simulink model "ims_Build5pt1g_tj"  (R2020b)
settings: Solver=FixedStepDiscrete  StartTime=0.0  StopTime=180  FixedStep=fem.Ts  RelTol=1e-4
InitFcn:
  | %
  | % Initialization callback function
  | %
  | 
  | try
  |    fprintf('\n New GMT IMS version!\n');
  | 
  |    % Get Simulink model directory
  |    [filepath,name,ext] = fileparts(which(bdroot));
  | 
  |    if ~strcmp(filepath,pwd)
  |       fprintf('\n Changing current directory to \n %s \n',filepath);
  |       cd(filepath);
  |    end
  | 
  |    %
  |    if(~exist('IMLoads','var'))
  |        warning('Simulation model assumes wind load is loaded...');
  |    end
  | catch
  |    warning('Running the InitFcn from puSimulate script');
  | end
values from neighbouring files (symbols this model uses):
  az = zeros(N,1)    [eval_trajectories.m]
  az_ff_en = 1    [load_IMS_5pt1g_tj.m]    (also in load_IMS_5pt1h_tj.m = 0)
  el = az    [eval_trajectories.m]
  el_ff_en = 1    [load_IMS_5pt1g_tj.m]    (also in load_IMS_5pt1h_tj.m = 0)
  fem =     [controls_5pt1g1K_z00_llTT_oad.mat]    (also in controls_5pt1g1K_z30_llTT_oad.mat)
  FEM_Ts = 1/1e3    (= 0.001)    [load_IMS_5pt1g_tj.m]    (also in load_IMS_5pt1h_tj.m)
  gir = az    [eval_trajectories.m]
  gir_ff_en = 1    [load_IMS_5pt1g_tj.m]    (also in load_IMS_5pt1h_tj.m = 0)
  H_tj = tf(1,[2*pi*0.1, 1])    [eval_trajectories.m]    (also in load_IMS_5pt1g_tj.m = c2d(Htjf,FEM_Ts, 'foh'); load_IMS_5pt1h_tj.m = c2d(Htjf,FEM_Ts, 'foh'))
  Hkin_fsm = Phi(fsm_out,1:3) * Phi_mnt_pinv    [compute_Hkin.m]
  Hkin_hp = Phi(hp_out,1:3) * Phi_mnt_pinv    [compute_Hkin.m]
  Hkin_m12 = [Phi(m1_out,1:3); Phi(m2_out,1:3)] * Phi_mnt_pinv    [compute_Hkin.m]    (also in eval_tjs.m = [Phi(m1_out,1:3); Phi(m2_out,1:3)] * pinv(Phi_mnt_enc))
  Hkin_m2p = Phi(m2p_out,1:3) * Phi_mnt_pinv    [compute_Hkin.m]
  Hkin_pmtnodes = Phi(pmt_out,1:3) * Phi_mnt_pinv    [compute_Hkin.m]    (also in eval_tjs.m = Phi(pmt_out,1:3) * pinv(Phi_mnt_enc))
  m1olf_en = 0    [load_IMS_5pt1g_tj.m]    (also in load_IMS_5pt1h_tj.m)
  m1sys =     [controls_5pt1g1K_z00_llTT_oad.mat]    (also in controls_5pt1g1K_z30_llTT_oad.mat)
  m2_pos_en = 0    [load_IMS_5pt1g_tj.m]    (also in load_IMS_5pt1h_tj.m)
  m2pos =     [controls_5pt1g1K_z00_llTT_oad.mat]    (also in controls_5pt1g1K_z30_llTT_oad.mat)
  m2pzt =     [controls_5pt1g1K_z00_llTT_oad.mat]    (also in controls_5pt1g1K_z30_llTT_oad.mat)
  m2PZT_en = 0    [load_IMS_5pt1g_tj.m]    (also in load_IMS_5pt1h_tj.m)
  mntFBc_en = 1    [load_IMS_5pt1g_tj.m]    (also in load_IMS_5pt1h_tj.m)
  mount =     [controls_5pt1g1K_z00_llTT_oad.mat]    (also in controls_5pt1g1K_z30_llTT_oad.mat; eval_tjs.m = mountY)
  om2 = (2*pi*eigenfrequencies).^2    [load_IMS_5pt1g_tj.m]    (also in load_IMS_5pt1h_tj.m)
  PG = zeros(length(om2),6)    [load_IMS_5pt1g_tj.m]    (also in load_IMS_5pt1h_tj.m)
  phiB = Phim(indDesInputs,:)'    [load_IMS_5pt1g_tj.m]    (also in load_IMS_5pt1h_tj.m)
  phiC = Phi(indDesOutputs,:)    [load_IMS_5pt1g_tj.m]    (also in load_IMS_5pt1h_tj.m)
  pmt1 = dlmread(pmt1_fname,',',[14,3,27,302])    [eval_tjs.m]    (also in eval_tjs_rtf_variants.m; load_IMS_5pt1g_tj.m; load_IMS_5pt1h_tj.m)
  pmt2 = dlmread(pmt2_fname,',',[14,3,10,302])    [eval_tjs.m]    (also in eval_tjs_rtf_variants.m; load_IMS_5pt1g_tj.m; load_IMS_5pt1h_tj.m)
  Psi_ss = gainMatrix(indDesOutputs,indDesInputs) - K_ss    [load_IMS_5pt1g_tj.m]    (also in load_IMS_5pt1h_tj.m)
  Psi_ssTs = 1/1000    (= 0.001)    [load_IMS_5pt1g_tj.m]    (also in load_IMS_5pt1h_tj.m)
  twice_zom = adjDamp*twice_zom    [load_IMS_5pt1g_tj.m]    (also in load_IMS_5pt1h_tj.m)
undefined symbols (not defined in the file or in its folder): DiscIntNeverNeededParam, magnitude
libraries: ims_block_library x20, simulink x1
(part 2 of 2)

== system ims_Build5pt1g_tj/M2_PZT_Control/PZT_Control_FSM3 ==
  PZT_cmd : Inport
  PZT_FB : Inport  Port=2
  Sum : Sum  Inputs=|+-
  multi-rate SS : ims_block_library/multi-rate SS  ss_model=m2pzt{3}.SSdtHfb
  rel_PZT_D : Gain  Gain=kron(eye(3),[-1,1])  Multiplication=Matrix(K*u)
  spliF_matrix : Gain  Gain=kron(eye(3),[-1;1])  Multiplication=Matrix(K*u)
  m2PZT_u : Outport  VectorParamsAs1DForOutWhenUnconnected=off
  wires:
  Sum/1 -> multi-rate SS/1
  spliF_matrix/1 -> m2PZT_u/1
  PZT_FB/1 -> rel_PZT_D/1
  rel_PZT_D/1 -> Sum/2
  PZT_cmd/1 -> Sum/1
  multi-rate SS/1 -> spliF_matrix/1

== system ims_Build5pt1g_tj/M2_PZT_Control/PZT_Control_FSM4 ==
  PZT_cmd : Inport
  PZT_FB : Inport  Port=2
  Sum : Sum  Inputs=|+-
  multi-rate SS : ims_block_library/multi-rate SS  ss_model=m2pzt{4}.SSdtHfb
  rel_PZT_D : Gain  Gain=kron(eye(3),[-1,1])  Multiplication=Matrix(K*u)
  spliF_matrix : Gain  Gain=kron(eye(3),[-1;1])  Multiplication=Matrix(K*u)
  m2PZT_u : Outport  VectorParamsAs1DForOutWhenUnconnected=off
  wires:
  Sum/1 -> multi-rate SS/1
  spliF_matrix/1 -> m2PZT_u/1
  PZT_FB/1 -> rel_PZT_D/1
  rel_PZT_D/1 -> Sum/2
  PZT_cmd/1 -> Sum/1
  multi-rate SS/1 -> spliF_matrix/1

== system ims_Build5pt1g_tj/M2_PZT_Control/PZT_Control_FSM5 ==
  PZT_cmd : Inport
  PZT_FB : Inport  Port=2
  Sum : Sum  Inputs=|+-
  multi-rate SS : ims_block_library/multi-rate SS  ss_model=m2pzt{5}.SSdtHfb
  rPZT : Scope
  rel_PZT_D : Gain  Gain=kron(eye(3),[-1,1])  Multiplication=Matrix(K*u)
  spliF_matrix : Gain  Gain=kron(eye(3),[-1;1])  Multiplication=Matrix(K*u)
  m2PZT_u : Outport  VectorParamsAs1DForOutWhenUnconnected=off
  wires:
  Sum/1 -> rPZT/1, multi-rate SS/1
  spliF_matrix/1 -> m2PZT_u/1
  PZT_FB/1 -> rel_PZT_D/1
  rel_PZT_D/1 -> Sum/2
  PZT_cmd/1 -> Sum/1
  multi-rate SS/1 -> spliF_matrix/1

== system ims_Build5pt1g_tj/M2_PZT_Control/PZT_Control_FSM6 ==
  PZT_cmd : Inport
  PZT_FB : Inport  Port=2
  Sum : Sum  Inputs=|+-
  multi-rate SS : ims_block_library/multi-rate SS  ss_model=m2pzt{6}.SSdtHfb
  rel_PZT_D : Gain  Gain=kron(eye(3),[-1,1])  Multiplication=Matrix(K*u)
  spliF_matrix : Gain  Gain=kron(eye(3),[-1;1])  Multiplication=Matrix(K*u)
  m2PZT_u : Outport  VectorParamsAs1DForOutWhenUnconnected=off
  wires:
  Sum/1 -> multi-rate SS/1
  spliF_matrix/1 -> m2PZT_u/1
  PZT_FB/1 -> rel_PZT_D/1
  rel_PZT_D/1 -> Sum/2
  PZT_cmd/1 -> Sum/1
  multi-rate SS/1 -> spliF_matrix/1

== system ims_Build5pt1g_tj/M2_PZT_Control/PZT_Control_FSM7 ==
  PZT_cmd : Inport
  PZT_FB : Inport  Port=2
  Sum : Sum  Inputs=|+-
  multi-rate SS : ims_block_library/multi-rate SS  ss_model=m2pzt{7}.SSdtHfb
  rel_PZT_D : Gain  Gain=kron(eye(3),[-1,1])  Multiplication=Matrix(K*u)
  spliF_matrix : Gain  Gain=kron(eye(3),[-1;1])  Multiplication=Matrix(K*u)
  m2PZT_u : Outport  VectorParamsAs1DForOutWhenUnconnected=off
  wires:
  Sum/1 -> multi-rate SS/1
  spliF_matrix/1 -> m2PZT_u/1
  PZT_FB/1 -> rel_PZT_D/1
  rel_PZT_D/1 -> Sum/2
  PZT_cmd/1 -> Sum/1
  multi-rate SS/1 -> spliF_matrix/1

== system ims_Build5pt1g_tj/Mount_Drv_PDR2021/AZ DT Lugre Fr model ==
  vel : Inport
  Enable : EnablePort
  Constant : Constant  Value=frParStruct.iIsSig01Active
  Discrete-Time Integrator : DiscreteIntegrator  SampleTime=-1  ICPrevOutput=DiscIntNeverNeededParam  ICPrevScaledInput=DiscIntNeverNeededParam
  Sum : Sum  Inputs=+++
  g(v) : Subsystem
  sigma_0 : Gain  Gain=frParStruct.sigm0
  sigma_1 : Gain  Gain=frParStruct.sigm1
  sigma_v : Gain  Gain=frParStruct.sigmv
  v2z : Subsystem
  FrTorque : Outport  VectorParamsAs1DForOutWhenUnconnected=off
  wires:
  Discrete-Time Integrator/1 -> sigma_0/1, v2z/3(z)
  g(v)/1(g) -> v2z/2(g(v))
  sigma_v/1 -> Sum/3  "Viscose Friction"
  v2z/1(dz) -> Discrete-Time Integrator/1, sigma_1/1
  sigma_1/1 -> Sum/1
  sigma_0/1 -> Sum/2
  Sum/1 -> FrTorque/1
  vel/1 -> v2z/1(v), g(v)/1(v), sigma_v/1
  Constant/1 -> g(v)/Enable, v2z/Enable

== system ims_Build5pt1g_tj/Mount_Drv_PDR2021/EL DT Lugre Fr model ==
  vel : Inport
  Enable : EnablePort
  Constant : Constant  Value=frParStruct.iIsSig01Active
  Discrete-Time Integrator : DiscreteIntegrator  SampleTime=-1  ICPrevOutput=DiscIntNeverNeededParam  ICPrevScaledInput=DiscIntNeverNeededParam
  Sum : Sum  Inputs=+++
  To Workspace : ToWorkspace  VariableName=el_Ve  SampleTime=-1
  To Workspace1 : ToWorkspace  VariableName=el_To  SampleTime=-1
  g(v) : Subsystem
  sigma_0 : Gain  Gain=frParStruct.sigm0
  sigma_1 : Gain  Gain=frParStruct.sigm1
  sigma_v : Gain  Gain=frParStruct.sigmv
  v2z : Subsystem
  FrTorque : Outport  VectorParamsAs1DForOutWhenUnconnected=off
  wires:
  sigma_v/1 -> Sum/3  "Viscose Friction"
  vel/1 -> v2z/1(v), g(v)/1(v), To Workspace/1, sigma_v/1
  Constant/1 -> g(v)/Enable, v2z/Enable
  sigma_0/1 -> Sum/2
  g(v)/1(g) -> v2z/2(g(v))
  sigma_1/1 -> Sum/1
  Discrete-Time Integrator/1 -> sigma_0/1, v2z/3(z)
  v2z/1(dz) -> Discrete-Time Integrator/1, sigma_1/1
  Sum/1 -> To Workspace1/1, FrTorque/1

== system ims_Build5pt1g_tj/Mount_Drv_PDR2021/GIR DT Lugre Fr model ==
  vel : Inport
  Enable : EnablePort
  Discrete-Time Integrator : DiscreteIntegrator  SampleTime=-1  ICPrevOutput=DiscIntNeverNeededParam  ICPrevScaledInput=DiscIntNeverNeededParam
  Gain : Gain  Gain=frParStruct.iIsSig01Active
  Scope : Scope
  Sum : Sum  Inputs=+++
  To Workspace : ToWorkspace  VariableName=gir_Ve  SampleTime=-1
  To Workspace1 : ToWorkspace  VariableName=gir_To  SampleTime=-1
  g(v) : Subsystem
  sigma_0 : Gain  Gain=frParStruct.sigm0
  sigma_1 : Gain  Gain=frParStruct.sigm1
  sigma_v : Gain  Gain=frParStruct.sigmv
  v2z : Subsystem
  FrTorque : Outport  VectorParamsAs1DForOutWhenUnconnected=off
  wires:
  sigma_v/1 -> Sum/3  "Viscose Friction"
  vel/1 -> Gain/1, To Workspace/1, sigma_v/1
  sigma_0/1 -> Sum/2
  g(v)/1(g) -> v2z/2(g(v))
  Discrete-Time Integrator/1 -> sigma_0/1, v2z/3(z)
  v2z/1(dz) -> Discrete-Time Integrator/1, Scope/1, sigma_1/1
  Sum/1 -> To Workspace1/1, FrTorque/1
  sigma_1/1 -> Sum/1
  Gain/1 -> v2z/1(v), g(v)/1(v)

== system ims_Build5pt1g_tj/Mount_Drv_PDR2021/ODC CT LUGRE Fr model ==
  Az vel : Inport
  EL_vel : Inport  Port=2
  GIR vel : Inport  Port=3
  Constant2 : Constant
  Demux1 : Demux  Outputs=3
  Friction : Subsystem
  Mux7 : Mux  Inputs=3
  Az Fr To : Outport  VectorParamsAs1DForOutWhenUnconnected=off
  El Fr To : Outport  Port=2  VectorParamsAs1DForOutWhenUnconnected=off
  Gir Fr To : Outport  Port=3  VectorParamsAs1DForOutWhenUnconnected=off
  wires:
  Mux7/1 -> Friction/1(Vel)
  Demux1/2 -> El Fr To/1
  Demux1/1 -> Az Fr To/1
  Friction/1(FrictionTo) -> Demux1/1
  Constant2/1 -> Friction/Enable
  Demux1/3 -> Gir Fr To/1
  Az vel/1 -> Mux7/1
  EL_vel/1 -> Mux7/2
  GIR vel/1 -> Mux7/3

== system ims_Build5pt1g_tj/Mount_Drv_PDR2021/Parasitic torques model  ==
  Az_pos_drv : Inport
  El_pos_drv : Inport  Port=2
  Gir_pos_drv : Inport  Port=3
  Az_drv_to : Inport  Port=4
  El_drv_to : Inport  Port=5
  Gir_drv_to : Inport  Port=6
  AZ_Parasitic_Torque : Subsystem  mask{ParasiticModelStruc=mount.az.ParasiticTo}
      mask prompts: ParasiticModelStruc "Parasitic Torque Model Parameters Structure"
  EL_Parasitic_Torque : Subsystem  mask{ParasiticModelStruc=mount.el.ParasiticTo}
      mask prompts: ParasiticModelStruc "Parasitic Torque Model Parameters Structure"
  GIR_Parasitic_Torque : Subsystem  mask{ParasiticModelStruc=mount.gir.ParasiticTo, T_pretension=mount.gir.T_pretension}
      mask prompts: ParasiticModelStruc "Parasitic Torque Model Parameters Structure"; T_pretension "Pretension torque"
  Mux1 : Mux  Commented=on  Inputs=2
  Mux2 : Mux  Commented=on  Inputs=2
  Mux6 : Mux  Commented=on  Inputs=2
  ParTo_Scope : Scope  Commented=on  NumInputPorts=3
  Subsystem : Subsystem  Commented=on
  Az_Par_To : Outport  VectorParamsAs1DForOutWhenUnconnected=off
  El_Par_To : Outport  Port=2  VectorParamsAs1DForOutWhenUnconnected=off
  Gir_Par_To : Outport  Port=3  VectorParamsAs1DForOutWhenUnconnected=off
  wires:
  Az_drv_to/1 -> Subsystem/2(Az To), AZ_Parasitic_Torque/2(Drive_Torque)
  Gir_drv_to/1 -> Subsystem/6(Gir To), GIR_Parasitic_Torque/2(Drive_Torque)
  GIR_Parasitic_Torque/1(Parasitic_Torque) -> Gir_Par_To/1, Mux6/1
  Gir_pos_drv/1 -> Subsystem/5(Gir Pos), GIR_Parasitic_Torque/1(Drive_Pos)
  El_drv_to/1 -> Subsystem/4(El To), EL_Parasitic_Torque/2(Drive_Torque)
  Az_pos_drv/1 -> Subsystem/1(Az Pos), AZ_Parasitic_Torque/1(Drive_Pos)
  El_pos_drv/1 -> Subsystem/3(El Pos), EL_Parasitic_Torque/1(Drive_Pos)
  AZ_Parasitic_Torque/1(Parasitic_Torque) -> Mux2/1, Az_Par_To/1
  EL_Parasitic_Torque/1(Parasitic_Torque) -> El_Par_To/1, Mux1/1
  Mux2/1 -> ParTo_Scope/1
  Mux1/1 -> ParTo_Scope/2
  Mux6/1 -> ParTo_Scope/3
  Subsystem/1(Out1) -> Mux2/2
  Subsystem/2(Out2) -> Mux1/2
  Subsystem/3(Out3) -> Mux6/2

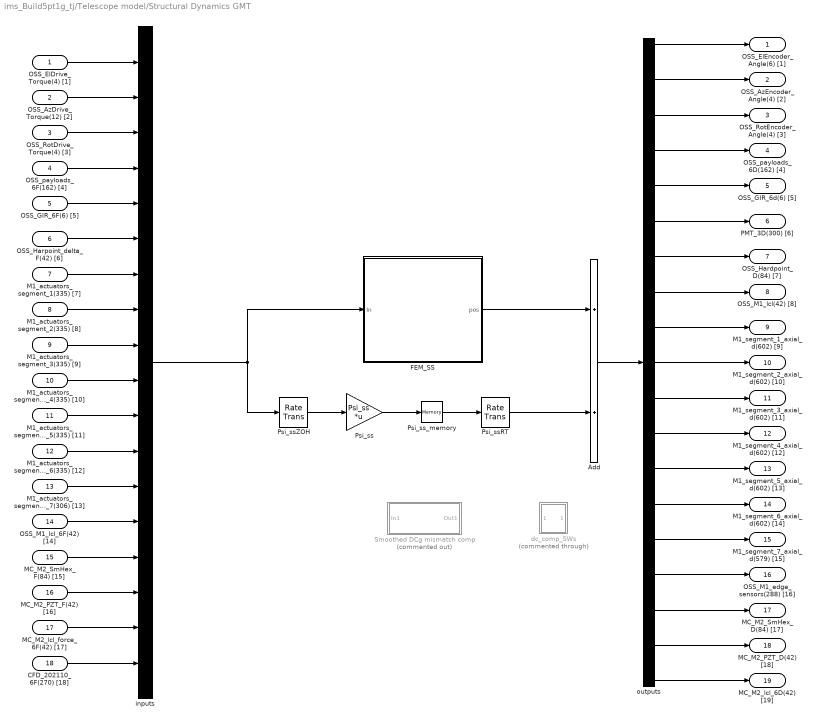
== system ims_Build5pt1g_tj/Telescope model/Structural Dynamics GMT ==
  OSS_ElDrive_Torque(4) [1] : Inport  PortDimensions=4
  OSS_AzDrive_Torque(12) [2] : Inport  Port=2  PortDimensions=12
  OSS_RotDrive_Torque(4) [3] : Inport  Port=3  PortDimensions=4
  OSS_payloads_6F(162) [4] : Inport  Port=4  PortDimensions=162
  OSS_GIR_6F(6) [5] : Inport  Port=5  PortDimensions=6
  OSS_Harpoint_delta_F(42) [6] : Inport  Port=6  PortDimensions=42
  M1_actuators_segment_1(335) [7] : Inport  Port=7  PortDimensions=335
  M1_actuators_segment_2(335) [8] : Inport  Port=8  PortDimensions=335
  M1_actuators_segment_3(335) [9] : Inport  Port=9  PortDimensions=335
  M1_actuators_segment_4(335) [10] : Inport  Port=10  PortDimensions=335
  M1_actuators_segment_5(335) [11] : Inport  Port=11  PortDimensions=335
  M1_actuators_segment_6(335) [12] : Inport  Port=12  PortDimensions=335
  M1_actuators_segment_7(306) [13] : Inport  Port=13  PortDimensions=306
  OSS_M1_lcl_6F(42) [14] : Inport  Port=14  PortDimensions=42
  MC_M2_SmHex_F(84) [15] : Inport  Port=15  PortDimensions=84
  MC_M2_PZT_F(42) [16] : Inport  Port=16  PortDimensions=42
  MC_M2_lcl_force_6F(42) [17] : Inport  Port=17  PortDimensions=42
  CFD_202110_6F(270) [18] : Inport  Port=18  PortDimensions=270
  Add : Sum
  FEM_SS : Subsystem
  Psi_ss : Gain  Gain=Psi_ss  Multiplication=Matrix(K*u) (u vector)
  Psi_ssRT : RateTransition  Deterministic=off  OutPortSampleTimeOpt=Inherit
  Psi_ssZOH : RateTransition  Deterministic=off  OutPortSampleTime=Psi_ssTs
  Psi_ss_memory : Memory  InitialCondition=zeros(size(phiC,1),1)  InheritSampleTime=on  LinearizeAsDelay=on
  Smoothed DCg mismatch comp : Subsystem  Commented=on
  dc_comp_SWs : Subsystem  Commented=through
  inputs : Mux  Inputs=modelMuxDims
  outputs : Demux  Outputs=modelDemuxDims
  OSS_ElEncoder_Angle(6) [1] : Outport  PortDimensions=6  VectorParamsAs1DForOutWhenUnconnected=off
  OSS_AzEncoder_Angle(4) [2] : Outport  Port=2  PortDimensions=4  VectorParamsAs1DForOutWhenUnconnected=off
  OSS_RotEncoder_Angle(4) [3] : Outport  Port=3  PortDimensions=4  VectorParamsAs1DForOutWhenUnconnected=off
  OSS_payloads_6D(162) [4] : Outport  Port=4  PortDimensions=162  VectorParamsAs1DForOutWhenUnconnected=off
  OSS_GIR_6d(6) [5] : Outport  Port=5  PortDimensions=6  VectorParamsAs1DForOutWhenUnconnected=off
  PMT_3D(300) [6] : Outport  Port=6  PortDimensions=300  VectorParamsAs1DForOutWhenUnconnected=off
  OSS_Hardpoint_D(84) [7] : Outport  Port=7  PortDimensions=84  VectorParamsAs1DForOutWhenUnconnected=off
  OSS_M1_lcl(42) [8] : Outport  Port=8  PortDimensions=42  VectorParamsAs1DForOutWhenUnconnected=off
  M1_segment_1_axial_d(602) [9] : Outport  Port=9  PortDimensions=602  VectorParamsAs1DForOutWhenUnconnected=off
  M1_segment_2_axial_d(602) [10] : Outport  Port=10  PortDimensions=602  VectorParamsAs1DForOutWhenUnconnected=off
  M1_segment_3_axial_d(602) [11] : Outport  Port=11  PortDimensions=602  VectorParamsAs1DForOutWhenUnconnected=off
  M1_segment_4_axial_d(602) [12] : Outport  Port=12  PortDimensions=602  VectorParamsAs1DForOutWhenUnconnected=off
  M1_segment_5_axial_d(602) [13] : Outport  Port=13  PortDimensions=602  VectorParamsAs1DForOutWhenUnconnected=off
  M1_segment_6_axial_d(602) [14] : Outport  Port=14  PortDimensions=602  VectorParamsAs1DForOutWhenUnconnected=off
  M1_segment_7_axial_d(579) [15] : Outport  Port=15  PortDimensions=579  VectorParamsAs1DForOutWhenUnconnected=off
  OSS_M1_edge_sensors(288) [16] : Outport  Port=16  PortDimensions=288  VectorParamsAs1DForOutWhenUnconnected=off
  MC_M2_SmHex_D(84) [17] : Outport  Port=17  PortDimensions=84  VectorParamsAs1DForOutWhenUnconnected=off
  MC_M2_PZT_D(42) [18] : Outport  Port=18  PortDimensions=42  VectorParamsAs1DForOutWhenUnconnected=off
  MC_M2_lcl_6D(42) [19] : Outport  Port=19  PortDimensions=42  VectorParamsAs1DForOutWhenUnconnected=off
  wires:
  outputs/19 -> MC_M2_lcl_6D(42) [19]/1
  outputs/18 -> MC_M2_PZT_D(42) [18]/1
  outputs/17 -> MC_M2_SmHex_D(84) [17]/1
  outputs/16 -> OSS_M1_edge_sensors(288) [16]/1
  outputs/15 -> M1_segment_7_axial_d(579) [15]/1
  outputs/14 -> M1_segment_6_axial_d(602) [14]/1
  outputs/13 -> M1_segment_5_axial_d(602) [13]/1
  outputs/12 -> M1_segment_4_axial_d(602) [12]/1
  outputs/11 -> M1_segment_3_axial_d(602) [11]/1
  outputs/10 -> M1_segment_2_axial_d(602) [10]/1
  outputs/9 -> M1_segment_1_axial_d(602) [9]/1
  outputs/8 -> OSS_M1_lcl(42) [8]/1
  outputs/7 -> OSS_Hardpoint_D(84) [7]/1
  outputs/6 -> PMT_3D(300) [6]/1
  outputs/5 -> OSS_GIR_6d(6) [5]/1
  outputs/4 -> OSS_payloads_6D(162) [4]/1
  outputs/3 -> OSS_RotEncoder_Angle(4) [3]/1
  outputs/2 -> OSS_AzEncoder_Angle(4) [2]/1
  outputs/1 -> OSS_ElEncoder_Angle(6) [1]/1
  CFD_202110_6F(270) [18]/1 -> inputs/18
  MC_M2_lcl_force_6F(42) [17]/1 -> inputs/17
  MC_M2_PZT_F(42) [16]/1 -> inputs/16
  MC_M2_SmHex_F(84) [15]/1 -> inputs/15
  OSS_M1_lcl_6F(42) [14]/1 -> inputs/14
  M1_actuators_segment_7(306) [13]/1 -> inputs/13
  M1_actuators_segment_6(335) [12]/1 -> inputs/12
  M1_actuators_segment_5(335) [11]/1 -> inputs/11
  M1_actuators_segment_4(335) [10]/1 -> inputs/10
  M1_actuators_segment_3(335) [9]/1 -> inputs/9
  M1_actuators_segment_2(335) [8]/1 -> inputs/8
  M1_actuators_segment_1(335) [7]/1 -> inputs/7
  OSS_Harpoint_delta_F(42) [6]/1 -> inputs/6
  OSS_GIR_6F(6) [5]/1 -> inputs/5
  OSS_payloads_6F(162) [4]/1 -> inputs/4
  OSS_RotDrive_Torque(4) [3]/1 -> inputs/3
  OSS_AzDrive_Torque(12) [2]/1 -> inputs/2
  OSS_ElDrive_Torque(4) [1]/1 -> inputs/1
  Psi_ss/1 -> Psi_ss_memory/1
  Add/1 -> outputs/1
  Psi_ssZOH/1 -> Psi_ss/1
  FEM_SS/1(pos) -> Add/1
  inputs/1 -> FEM_SS/1(In), Psi_ssZOH/1
  Psi_ss_memory/1 -> Psi_ssRT/1
  Psi_ssRT/1 -> Add/2

== system ims_Build5pt1g_tj/Mount_Drv_PDR2021/AZ DT Lugre Fr model/g(v) ==
  v : Inport
  Enable : EnablePort
  Constant : Constant  Value=0
  gs : Subsystem
  g : Outport  VectorParamsAs1DForOutWhenUnconnected=off
  wires:
  gs/1(gs(v)) -> g/1
  v/1 -> gs/1(v)
  Constant/1 -> gs/Enable

== system ims_Build5pt1g_tj/Mount_Drv_PDR2021/AZ DT Lugre Fr model/v2z ==
  v : Inport
  g(v) : Inport  Port=2
  z : Inport  Port=3
  Enable : EnablePort
  Abs : Abs
  Divide : Product  Inputs=*/*
  Sum : Sum  Inputs=|+-
  dz : Outport  VectorParamsAs1DForOutWhenUnconnected=off
  wires:
  Abs/1 -> Divide/1
  Divide/1 -> Sum/2
  v/1 -> Sum/1, Abs/1
  Sum/1 -> dz/1
  g(v)/1 -> Divide/2
  z/1 -> Divide/3

== system ims_Build5pt1g_tj/Mount_Drv_PDR2021/EL DT Lugre Fr model/g(v) ==
  v : Inport
  Enable : EnablePort
  Constant : Constant  Value=0
  Sum : Sum  Inputs=|++
  gc : Constant  Value=frParStruct.Tc/frParStruct.sigm0
  gs : Subsystem
  g : Outport  VectorParamsAs1DForOutWhenUnconnected=off
  wires:
  Sum/1 -> g/1
  v/1 -> gs/1(v)
  gs/1(gs(v)) -> Sum/1
  Constant/1 -> gs/Enable
  gc/1 -> Sum/2

== system ims_Build5pt1g_tj/Mount_Drv_PDR2021/EL DT Lugre Fr model/v2z ==
  v : Inport
  g(v) : Inport  Port=2
  z : Inport  Port=3
  Enable : EnablePort
  Abs : Abs
  Divide : Product  Inputs=*/*
  Sum : Sum  Inputs=|+-
  dz : Outport  VectorParamsAs1DForOutWhenUnconnected=off
  wires:
  Abs/1 -> Divide/1
  Divide/1 -> Sum/2
  v/1 -> Sum/1, Abs/1
  Sum/1 -> dz/1
  g(v)/1 -> Divide/2
  z/1 -> Divide/3

== system ims_Build5pt1g_tj/Mount_Drv_PDR2021/GIR DT Lugre Fr model/g(v) ==
  v : Inport
  Constant : Constant  Value=0
  Sum : Sum  Inputs=|++
  gc : Constant  Value=frParStruct.Tc/frParStruct.sigm0
  gs : Subsystem
  g : Outport  VectorParamsAs1DForOutWhenUnconnected=off
  wires:
  Sum/1 -> g/1
  v/1 -> gs/1(v)
  gs/1(gs(v)) -> Sum/1
  gc/1 -> Sum/2
  Constant/1 -> gs/Enable

== system ims_Build5pt1g_tj/Mount_Drv_PDR2021/GIR DT Lugre Fr model/v2z ==
  v : Inport
  g(v) : Inport  Port=2
  z : Inport  Port=3
  Abs : Abs
  Divide : Product  Inputs=*/*
  Sum : Sum  Inputs=|+-
  dz : Outport  VectorParamsAs1DForOutWhenUnconnected=off
  wires:
  Abs/1 -> Divide/1
  Divide/1 -> Sum/2
  v/1 -> Sum/1, Abs/1
  Sum/1 -> dz/1
  g(v)/1 -> Divide/2
  z/1 -> Divide/3

== system ims_Build5pt1g_tj/Mount_Drv_PDR2021/ODC CT LUGRE Fr model/Friction ==
  Vel : Inport
  Enable : EnablePort
  Constant : Constant  Value=az.oFr.iIsActive
  Constant1 : Constant  Value=el.oFr.iIsActive
  Constant2 : Constant  Value=gir.oFr.iIsActive
  Demux1 : Demux  Outputs=3
  Friction Alt : Subsystem  mask{sigma0=el.oFr.sigm0, sigma1=el.oFr.sigm1, Tc=el.oFr.Tc, sigmav=el.oFr.sigmv, Ts=el.oFr.Ts, vs=el.oFr.vs, iIsSig01Active=el.oFr.iIsSig01Active}
      mask prompts: iIsSig01Active "0=inactive, 1=active"
  Friction Az : Subsystem  mask{sigma0=az.oFr.sigm0, sigma1=az.oFr.sigm1, Tc=az.oFr.Tc, sigmav=az.oFr.sigmv, Ts=az.oFr.Ts, vs=az.oFr.vs, iIsSig01Active=az.oFr.iIsSig01Active}
      mask prompts: iIsSig01Active "0=inactive, 1=active"
  Friction Gir : Subsystem  mask{sigma0=gir.oFr.sigm0, sigma1=gir.oFr.sigm1, Tc=gir.oFr.Tc, sigmav=gir.oFr.sigmv, Ts=gir.oFr.Ts, vs=gir.oFr.vs, iIsSig01Active=gir.oFr.iIsSig01Active}
      mask prompts: iIsSig01Active "0=inactive, 1=active"
  Mux2 : Mux  Inputs=3
  FrictionTo : Outport
  wires:
  Friction Alt/1(Tfr) -> Mux2/2
  Demux1/2 -> Friction Alt/1(v)
  Vel/1 -> Demux1/1
  Demux1/1 -> Friction Az/1(v)
  Friction Az/1(Tfr) -> Mux2/1
  Mux2/1 -> FrictionTo/1
  Constant1/1 -> Friction Alt/Enable
  Constant/1 -> Friction Az/Enable
  Constant2/1 -> Friction Gir/Enable
  Demux1/3 -> Friction Gir/1(v)
  Friction Gir/1(Tfr) -> Mux2/3

== system ims_Build5pt1g_tj/Mount_Drv_PDR2021/Parasitic torques model /AZ_Parasitic_Torque ==
  Drive_Pos : Inport
  Drive_Torque : Inport  Port=2
  Cogging : Lookup_n-D  NumberOfTableDimensions=1  LookupTableObject=F_ripple  BreakpointsForDimension1=ParasiticModelStruc.Pos  Table=ParasiticModelStruc.oCog.Amp  InternalRulePriority=Speed  RndMeth=Simplest  InputSameDT=on
  Constant : Constant  Value=0.1869
  Divide : Product  Inputs=**
  EMF Distortion : Lookup_n-D  NumberOfTableDimensions=1  LookupTableObject=F_ripple  BreakpointsForDimension1=ParasiticModelStruc.Pos  Table=ParasiticModelStruc.oEmf.Amp  InternalRulePriority=Speed  RndMeth=Simplest  InputSameDT=on
  Gain : Gain  Gain=1/ParasiticModelStruc.R
  Gain1 : Gain  Gain=1/250
  Gain2 : Gain  Gain=1/ParasiticModelStruc.N_Segm
  Mod : Math  Operator=rem  SignedPower=on  SaturateOnIntegerOverflow=on
  Mod1 : Math  Operator=rem  SignedPower=on  SaturateOnIntegerOverflow=on
  Radius : Gain  Gain=ParasiticModelStruc.R
  Sum1 : Sum
  Sum2 : Sum
  Parasitic_Torque : Outport  VectorParamsAs1DForOutWhenUnconnected=off
  wires:
  Divide/1 -> Sum1/1
  Gain1/1 -> Gain2/1  "I_rms"
  Mod1/1 -> EMF Distortion/1, Cogging/1
  Cogging/1 -> Sum1/2
  Radius/1 -> Mod/1  "driven  distance"
  Drive_Torque/1 -> Gain/1
  Gain/1 -> Gain1/1  "Force"
  EMF Distortion/1 -> Divide/2
  Sum2/1 -> Mod1/1
  Mod/1 -> Sum2/1
  Gain2/1 -> Divide/1  "I_rms pro Segment"
  Constant/1 -> Mod/2, Sum2/2, Mod1/2
  Drive_Pos/1 -> Radius/1  "Drive Position"
  Sum1/1 -> Parasitic_Torque/1

== system ims_Build5pt1g_tj/Mount_Drv_PDR2021/Parasitic torques model /EL_Parasitic_Torque ==
  Drive_Pos : Inport
  Drive_Torque : Inport  Port=2
  Cogging : Lookup_n-D  NumberOfTableDimensions=1  LookupTableObject=F_ripple  BreakpointsForDimension1=ParasiticModelStruc.Pos  Table=ParasiticModelStruc.oCog.Amp  InternalRulePriority=Speed  RndMeth=Simplest  InputSameDT=on
  Constant : Constant  Value=0.1869
  Divide : Product  Inputs=**
  EMF Distortion : Lookup_n-D  NumberOfTableDimensions=1  LookupTableObject=F_ripple  BreakpointsForDimension1=ParasiticModelStruc.Pos  Table=ParasiticModelStruc.oEmf.Amp  InternalRulePriority=Speed  RndMeth=Simplest  InputSameDT=on
  Gain : Gain  Gain=1/ParasiticModelStruc.R
  Gain1 : Gain  Gain=1/250
  Gain2 : Gain  Gain=1/ParasiticModelStruc.N_Segm
  Mod : Math  Operator=rem  SignedPower=on  SaturateOnIntegerOverflow=on
  Mod1 : Math  Operator=rem  SignedPower=on  SaturateOnIntegerOverflow=on
  Radius : Gain  Gain=ParasiticModelStruc.R
  Sum1 : Sum
  Sum2 : Sum
  Parasitic_Torque : Outport  VectorParamsAs1DForOutWhenUnconnected=off
  wires:
  Sum1/1 -> Parasitic_Torque/1
  Drive_Torque/1 -> Gain/1
  EMF Distortion/1 -> Divide/2
  Drive_Pos/1 -> Radius/1  "Drive Position"
  Gain1/1 -> Gain2/1  "I_rms"
  Gain2/1 -> Divide/1  "I_rms pro Segment"
  Gain/1 -> Gain1/1  "Force"
  Mod/1 -> Sum2/1
  Cogging/1 -> Sum1/2
  Radius/1 -> Mod/1  "driven  distance"
  Sum2/1 -> Mod1/1
  Mod1/1 -> EMF Distortion/1, Cogging/1
  Divide/1 -> Sum1/1
  Constant/1 -> Mod/2, Sum2/2, Mod1/2

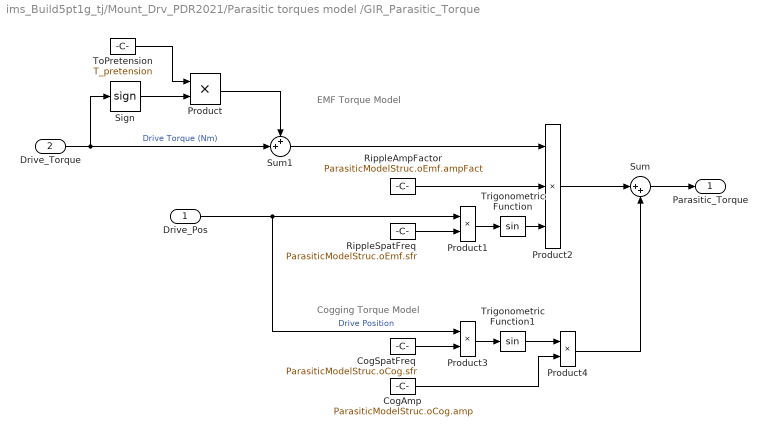
== system ims_Build5pt1g_tj/Mount_Drv_PDR2021/Parasitic torques model /GIR_Parasitic_Torque ==
  note: EMF Torque Model
  note: Cogging Torque Model
  Drive_Pos : Inport
  Drive_Torque : Inport  Port=2
  CogAmp : Constant  Value=ParasiticModelStruc.oCog.amp
  CogSpatFreq : Constant  Value=ParasiticModelStruc.oCog.sfr
  Product : Product
  Product1 : Product  RndMeth=Zero
  Product2 : Product  Inputs=3  RndMeth=Zero
  Product3 : Product  RndMeth=Zero
  Product4 : Product  RndMeth=Zero
  RippleAmpFactor : Constant  Value=ParasiticModelStruc.oEmf.ampFact
  RippleSpatFreq : Constant  Value=ParasiticModelStruc.oEmf.sfr
  Sign : Signum
  Sum : Sum  Inputs=|++
  Sum1 : Sum  Inputs=++|
  ToPretension : Constant  Value=T_pretension
  Trigonometric Function : Trigonometry
  Trigonometric Function1 : Trigonometry
  Parasitic_Torque : Outport  VectorParamsAs1DForOutWhenUnconnected=off
  wires:
  RippleAmpFactor/1 -> Product2/2
  Product1/1 -> Trigonometric Function/1
  RippleSpatFreq/1 -> Product1/2
  Product3/1 -> Trigonometric Function1/1
  Trigonometric Function1/1 -> Product4/1
  CogSpatFreq/1 -> Product3/2
  Drive_Pos/1 -> Product3/1, Product1/1  "Drive Position"
  CogAmp/1 -> Product4/2
  Product4/1 -> Sum/2
  Product2/1 -> Sum/1
  Sum/1 -> Parasitic_Torque/1
  Trigonometric Function/1 -> Product2/3
  Sum1/1 -> Product2/1
  Drive_Torque/1 -> Sign/1, Sum1/2  "Drive Torque (Nm)"
  Sign/1 -> Product/2
  ToPretension/1 -> Product/1
  Product/1 -> Sum1/1

== system ims_Build5pt1g_tj/Mount_Drv_PDR2021/Parasitic torques model /Subsystem ==
  Az Pos : Inport
  Az To : Inport  Port=2
  El Pos : Inport  Port=3
  El To : Inport  Port=4
  Gir Pos : Inport  Port=5
  Gir To : Inport  Port=6
  Constant2 : Constant
  Demux1 : Demux  Outputs=3
  Mux1 : Mux  Inputs=3
  Mux7 : Mux  Inputs=3
  Parasitic Torques : Subsystem
  Out1 : Outport  VectorParamsAs1DForOutWhenUnconnected=off
  Out2 : Outport  Port=2  VectorParamsAs1DForOutWhenUnconnected=off
  Out3 : Outport  Port=3  VectorParamsAs1DForOutWhenUnconnected=off
  wires:
  Demux1/1 -> Out1/1
  Demux1/2 -> Out2/1
  Gir Pos/1 -> Mux7/3
  Demux1/3 -> Out3/1
  Az Pos/1 -> Mux7/1
  Mux7/1 -> Parasitic Torques/2(MotPos)
  Mux1/1 -> Parasitic Torques/1(MotTo)
  Constant2/1 -> Parasitic Torques/Enable
  El Pos/1 -> Mux7/2
  Parasitic Torques/1(ParasiticTo) -> Demux1/1
  Az To/1 -> Mux1/1
  El To/1 -> Mux1/2
  Gir To/1 -> Mux1/3

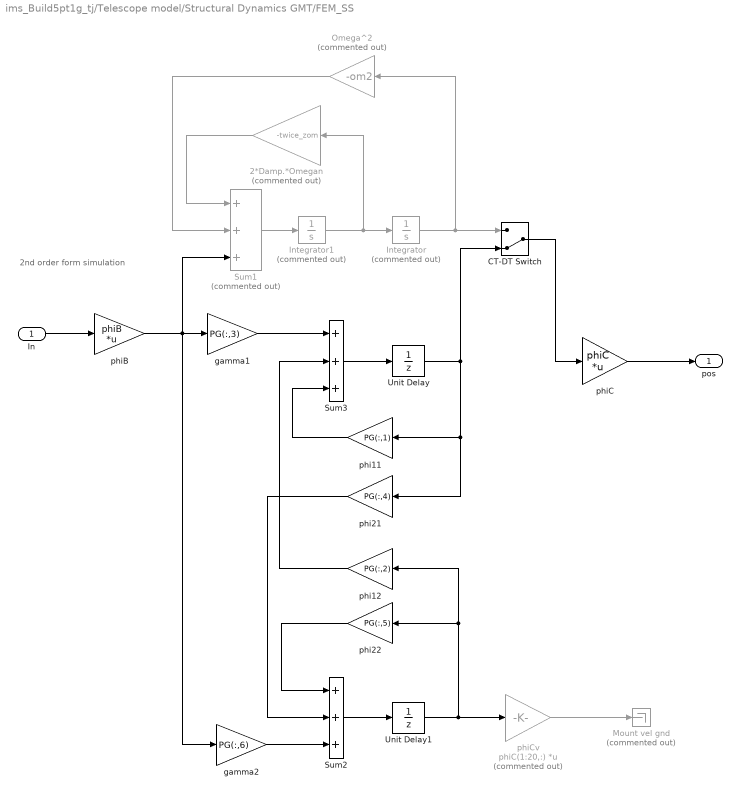
== system ims_Build5pt1g_tj/Telescope model/Structural Dynamics GMT/FEM_SS ==
  note: 2nd order form simulation
  In : Inport
  2*Damp.*Omegan : Gain  Commented=on  Gain=-twice_zom
  CT-DT Switch : ManualSwitch  CurrentSetting=0
  Integrator : Integrator  Commented=on
  Integrator1 : Integrator  Commented=on
  Mount vel gnd : Terminator  Commented=on
  Omega^2 : Gain  Commented=on  Gain=-om2
  Sum1 : Sum  Commented=on  Inputs=+++
  Sum2 : Sum  Inputs=+++
  Sum3 : Sum  Inputs=+++
  Unit Delay : UnitDelay  SampleTime=FEM_Ts  HasFrameUpgradeWarning=on
  Unit Delay1 : UnitDelay  SampleTime=FEM_Ts  HasFrameUpgradeWarning=on
  gamma1 : Gain  Gain=PG(:,3)
  gamma2 : Gain  Gain=PG(:,6)
  phi11 : Gain  Gain=PG(:,1)
  phi12 : Gain  Gain=PG(:,2)
  phi21 : Gain  Gain=PG(:,4)
  phi22 : Gain  Gain=PG(:,5)
  phiB : Gain  Gain=phiB  Multiplication=Matrix(K*u) (u vector)
  phiC : Gain  Gain=phiC  Multiplication=Matrix(K*u) (u vector)
  phiCv : Gain  Commented=on  Gain=phiC(1:20,:)  Multiplication=Matrix(K*u) (u vector)
  pos : Outport  VectorParamsAs1DForOutWhenUnconnected=off
  wires:
  Unit Delay/1 -> CT-DT Switch/2, phi11/1, phi21/1
  phi12/1 -> Sum3/2
  Sum2/1 -> Unit Delay1/1
  Sum3/1 -> Unit Delay/1
  gamma2/1 -> Sum2/3
  phi21/1 -> Sum2/2
  phi22/1 -> Sum2/1
  gamma1/1 -> Sum3/1
  phi11/1 -> Sum3/3
  Unit Delay1/1 -> phiCv/1, phi12/1, phi22/1
  phiB/1 -> Sum1/3, gamma2/1, gamma1/1
  phiC/1 -> pos/1
  In/1 -> phiB/1
  phiCv/1 -> Mount vel gnd/1
  Integrator1/1 -> Integrator/1, 2*Damp.*Omegan/1
  Omega^2/1 -> Sum1/2
  2*Damp.*Omegan/1 -> Sum1/1
  Sum1/1 -> Integrator1/1
  Integrator/1 -> CT-DT Switch/1, Omega^2/1
  CT-DT Switch/1 -> phiC/1

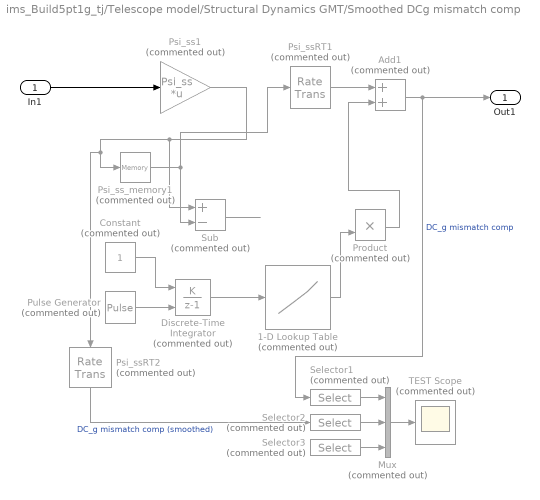
== system ims_Build5pt1g_tj/Telescope model/Structural Dynamics GMT/Smoothed DCg mismatch comp ==
  In1 : Inport
  1-D Lookup Table : Lookup_n-D  Commented=on  NumberOfTableDimensions=1  BreakpointsSpecification=Even spacing  IndexSearchMethod=Evenly spaced points  Table=shapeFilt(2:end)  InterpMethod=Nearest  DiagnosticForOutOfRangeInput=Warning  InternalRulePriority=Speed  RndMeth=Simplest  InputSameDT=on
  Add1 : Sum  Commented=on
  Constant : Constant  Commented=on
  Discrete-Time Integrator : DiscreteIntegrator  Commented=on  IntegratorMethod=Accumulation: Forward Euler  gainval=1  ExternalReset=rising  InitialCondition=1  SampleTime=-1  ICPrevOutput=DiscIntNeverNeededParam  ICPrevScaledInput=DiscIntNeverNeededParam
  Mux : Mux  Commented=on  Inputs=3
  Product : Product  Commented=on
  Psi_ss1 : Gain  Commented=on  Gain=Psi_ss  Multiplication=Matrix(K*u) (u vector)
  Psi_ssRT1 : RateTransition  Commented=on  OutPortSampleTimeOpt=Inherit
  Psi_ssRT2 : RateTransition  Commented=on  OutPortSampleTimeOpt=Inherit
  Psi_ss_memory1 : Memory  Commented=on  InitialCondition=zeros(size(phiC,1),1)  InheritSampleTime=on  LinearizeAsDelay=on
  Pulse Generator : DiscretePulseGenerator  Commented=on  Period=Psi_ssTs/fem.Ts  PulseWidth=2  SampleTime=fem.Ts
  Selector1 : Selector  Commented=on  InputPortWidth=size(phiC,1)  IndexOptions=Index vector (dialog)  Indices=[183]  OutputSizes=1
  Selector2 : Selector  Commented=on  InputPortWidth=size(phiC,1)  IndexOptions=Index vector (dialog)  Indices=[183]  OutputSizes=1
  Selector3 : Selector  Commented=on  InputPortWidth=size(phiC,1)  IndexOptions=Index vector (dialog)  Indices=[183]  OutputSizes=1
  Sub : Sum  Commented=on  Inputs=+-
  TEST Scope : Scope  Commented=on
  Out1 : Outport  VectorParamsAs1DForOutWhenUnconnected=off
  wires:
  Selector1/1 -> Mux/1
  Add1/1 -> Out1/1, Selector1/1  "DC_g mismatch comp"
  1-D Lookup Table/1 -> Product/2
  Pulse Generator/1 -> Discrete-Time Integrator/2
  Constant/1 -> Discrete-Time Integrator/1
  Psi_ssRT2/1 -> Selector2/1  "DC_g mismatch comp (smoothed)"
  Psi_ss1/1 -> Psi_ss_memory1/1, Psi_ssRT2/1, Sub/1
  Discrete-Time Integrator/1 -> 1-D Lookup Table/1
  Sub/1 -> ?
  Mux/1 -> TEST Scope/1
  Psi_ss_memory1/1 -> Sub/2, Psi_ssRT1/1
  Selector2/1 -> Mux/2
  Product/1 -> Add1/2
  Psi_ssRT1/1 -> Add1/1
  In1/1 -> Psi_ss1/1
  Selector3/1 -> Mux/3

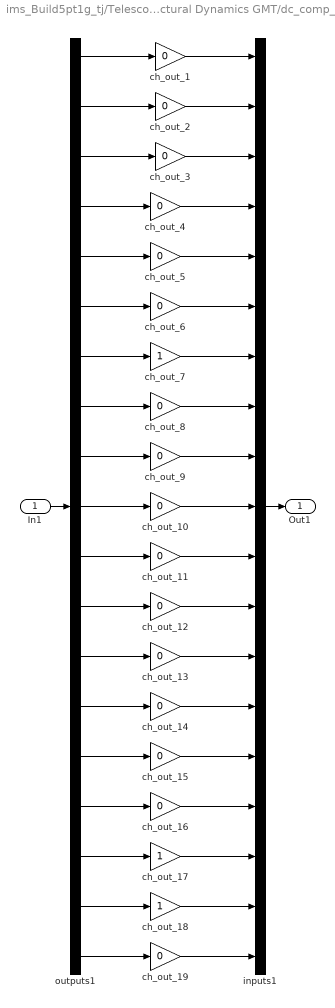
== system ims_Build5pt1g_tj/Telescope model/Structural Dynamics GMT/dc_comp_SWs ==
  In1 : Inport
  ch_out_{1..6,8..16,19} (16 alike) : Gain  Gain=0
  ch_out_17 : Gain
  ch_out_18 : Gain
  ch_out_7 : Gain
  inputs1 : Mux  Inputs=modelDemuxDims
  outputs1 : Demux  Outputs=modelDemuxDims
  Out1 : Outport
  wires:
  inputs1/1 -> Out1/1
  outputs1/1 -> ch_out_1/1
  ch_out_9/1 -> inputs1/9
  ch_out_14/1 -> inputs1/14
  ch_out_4/1 -> inputs1/4
  ch_out_18/1 -> inputs1/18
  ch_out_7/1 -> inputs1/7
  outputs1/6 -> ch_out_6/1
  ch_out_6/1 -> inputs1/6
  ch_out_10/1 -> inputs1/10
  ch_out_11/1 -> inputs1/11
  outputs1/16 -> ch_out_16/1
  outputs1/19 -> ch_out_19/1
  In1/1 -> outputs1/1
  ch_out_12/1 -> inputs1/12
  outputs1/8 -> ch_out_8/1
  outputs1/10 -> ch_out_10/1
  ch_out_5/1 -> inputs1/5
  ch_out_3/1 -> inputs1/3
  ch_out_19/1 -> inputs1/19
  ch_out_16/1 -> inputs1/16
  ch_out_2/1 -> inputs1/2
  ch_out_15/1 -> inputs1/15
  outputs1/18 -> ch_out_18/1
  ch_out_13/1 -> inputs1/13
  outputs1/2 -> ch_out_2/1
  outputs1/7 -> ch_out_7/1
  ch_out_8/1 -> inputs1/8
  outputs1/9 -> ch_out_9/1
  outputs1/5 -> ch_out_5/1
  outputs1/4 -> ch_out_4/1
  outputs1/14 -> ch_out_14/1
  outputs1/13 -> ch_out_13/1
  ch_out_1/1 -> inputs1/1
  ch_out_17/1 -> inputs1/17
  outputs1/12 -> ch_out_12/1
  outputs1/15 -> ch_out_15/1
  outputs1/17 -> ch_out_17/1
  outputs1/3 -> ch_out_3/1
  outputs1/11 -> ch_out_11/1

== system ims_Build5pt1g_tj/Mount_Drv_PDR2021/AZ DT Lugre Fr model/g(v)/gs ==
  v : Inport
  Enable : EnablePort
  Divide : Product  Inputs=**
  Gain : Gain  Gain=1/frParStruct.vs
  Math Function : Math  SignedPower=on  SaturateOnIntegerOverflow=on
  Math Function1 : Math  Operator=magnitude^2  SignedPower=on  SaturateOnIntegerOverflow=on
  Sum : Sum  Inputs=|++
  Unary Minus : UnaryMinus
  gc : Constant  Value=frParStruct.Tc/frParStruct.sigm0
  gs : Constant  Value=(frParStruct.Ts-frParStruct.Tc)/frParStruct.sigm0
  gs(v) : Outport  VectorParamsAs1DForOutWhenUnconnected=off
  wires:
  Math Function/1 -> Divide/1
  gs/1 -> Divide/2
  Math Function1/1 -> Unary Minus/1
  Unary Minus/1 -> Math Function/1
  Gain/1 -> Math Function1/1
  v/1 -> Gain/1
  gc/1 -> Sum/2
  Divide/1 -> Sum/1
  Sum/1 -> gs(v)/1

== system ims_Build5pt1g_tj/Mount_Drv_PDR2021/EL DT Lugre Fr model/g(v)/gs ==
  v : Inport
  Enable : EnablePort
  Divide : Product  Inputs=**
  Gain : Gain  Gain=1/frParStruct.vs
  Math Function : Math  SignedPower=on  SaturateOnIntegerOverflow=on
  Math Function1 : Math  Operator=magnitude^2  SignedPower=on  SaturateOnIntegerOverflow=on
  Unary Minus : UnaryMinus
  gs : Constant  Value=(frParStruct.Ts-frParStruct.Tc)/frParStruct.sigm0
  gs(v) : Outport  VectorParamsAs1DForOutWhenUnconnected=off
  wires:
  Math Function/1 -> Divide/1
  gs/1 -> Divide/2
  Math Function1/1 -> Unary Minus/1
  Unary Minus/1 -> Math Function/1
  Gain/1 -> Math Function1/1
  v/1 -> Gain/1
  Divide/1 -> gs(v)/1

== system ims_Build5pt1g_tj/Mount_Drv_PDR2021/GIR DT Lugre Fr model/g(v)/gs ==
  v : Inport
  Enable : EnablePort
  Divide : Product  Inputs=**
  Gain : Gain  Gain=1/frParStruct.vs
  Math Function : Math  SignedPower=on  SaturateOnIntegerOverflow=on
  Math Function1 : Math  Operator=magnitude^2  SignedPower=on  SaturateOnIntegerOverflow=on
  Unary Minus : UnaryMinus
  gs : Constant  Value=(frParStruct.Ts-frParStruct.Tc)/frParStruct.sigm0
  gs(v) : Outport  VectorParamsAs1DForOutWhenUnconnected=off
  wires:
  Math Function/1 -> Divide/1
  gs/1 -> Divide/2
  Math Function1/1 -> Unary Minus/1
  Unary Minus/1 -> Math Function/1
  Gain/1 -> Math Function1/1
  v/1 -> Gain/1
  Divide/1 -> gs(v)/1

== system ims_Build5pt1g_tj/Mount_Drv_PDR2021/ODC CT LUGRE Fr model/Friction/Friction Alt ==
  v : Inport
  Enable : EnablePort
  Constant : Constant  Value=iIsSig01Active
  Integrator2 : Integrator
  Sum : Sum  Inputs=+++
  g(v) : Subsystem
  sigma_0 : Gain  Gain=sigma0
  sigma_1 : Gain  Gain=sigma1
  sigma_v : Gain  Gain=sigmav
  v2z : Subsystem
  Tfr : Outport
  wires:
  v2z/1(dz) -> Integrator2/1, sigma_1/1
  Integrator2/1 -> sigma_0/1, v2z/3(z)
  g(v)/1(g) -> v2z/2(g(v))
  sigma_0/1 -> Sum/2
  Sum/1 -> Tfr/1
  sigma_1/1 -> Sum/1
  sigma_v/1 -> Sum/3
  v/1 -> g(v)/1(v), v2z/1(v), sigma_v/1
  Constant/1 -> v2z/Enable, g(v)/Enable

== system ims_Build5pt1g_tj/Mount_Drv_PDR2021/ODC CT LUGRE Fr model/Friction/Friction Az ==
  v : Inport
  Enable : EnablePort
  Constant : Constant  Value=iIsSig01Active
  Integrator2 : Integrator
  Sum : Sum  Inputs=+++
  g(v) : Subsystem
  sigma_0 : Gain  Gain=sigma0
  sigma_1 : Gain  Gain=sigma1
  sigma_v : Gain  Gain=sigmav
  v2z : Subsystem
  Tfr : Outport
  wires:
  v2z/1(dz) -> Integrator2/1, sigma_1/1
  Integrator2/1 -> sigma_0/1, v2z/3(z)
  g(v)/1(g) -> v2z/2(g(v))
  sigma_0/1 -> Sum/2
  Sum/1 -> Tfr/1
  sigma_1/1 -> Sum/1
  sigma_v/1 -> Sum/3
  v/1 -> g(v)/1(v), v2z/1(v), sigma_v/1
  Constant/1 -> g(v)/Enable, v2z/Enable

== system ims_Build5pt1g_tj/Mount_Drv_PDR2021/ODC CT LUGRE Fr model/Friction/Friction Gir ==
  v : Inport
  Enable : EnablePort
  Integrator2 : Integrator
  Sum : Sum  Inputs=+++
  g(v) : Subsystem
  iIsSig01Active : Gain  Gain=iIsSig01Active
  sigma_0 : Gain  Gain=sigma0
  sigma_1 : Gain  Gain=sigma1
  sigma_v : Gain  Gain=sigmav
  v2z : Subsystem
  Tfr : Outport
  wires:
  v2z/1(dz) -> Integrator2/1, sigma_1/1
  v/1 -> sigma_v/1, iIsSig01Active/1
  Integrator2/1 -> sigma_0/1, v2z/3(z)
  g(v)/1(g) -> v2z/2(g(v))
  sigma_0/1 -> Sum/2
  Sum/1 -> Tfr/1
  sigma_1/1 -> Sum/1
  sigma_v/1 -> Sum/3
  iIsSig01Active/1 -> g(v)/1(v), v2z/1(v)

== system ims_Build5pt1g_tj/Mount_Drv_PDR2021/Parasitic torques model /Subsystem/Parasitic Torques ==
  MotTo : Inport
  MotPos : Inport  Port=2
  Enable : EnablePort
  Demux1 : Demux  Outputs=2
  Demux2 : Demux  Outputs=2
  Demux3 : Demux  Outputs=2
  Mux2 : Mux  Inputs=2
  Mux3 : Mux  Inputs=3
  Parasitic AZ : Subsystem  mask{Pos=az.oParasitic.Pos, Amp_Cog=az.oParasitic.oCog.Amp, Amp_EMF=az.oParasitic.oEmf.Amp, R=az.oParasitic.R, N_Segm=az.oParasitic.N_Segm}
  Parasitic EL : Subsystem  mask{Pos=el.oParasitic.Pos, Amp_Cog=el.oParasitic.oCog.Amp, Amp_EMF=el.oParasitic.oEmf.Amp, R=el.oParasitic.R, N_Segm=el.oParasitic.N_Segm}
  Parasitic GIR : Subsystem  mask{cog_sfr=gir.oParasitic.oCog.sfr, cog_amp=gir.oParasitic.oCog.amp, emf_sfr=gir.oParasitic.oEmf.sfr, emf_ampFact=gir.oParasitic.oEmf.ampFact, T_pretension=gir.T_pretension}
  Sel : Selector  InputPortWidth=6  IndexOptions=Index vector (dialog)  Indices=[1 4]  OutputSizes=1
  Sel1 : Selector  InputPortWidth=6  IndexOptions=Index vector (dialog)  Indices=[2 5]  OutputSizes=1
  Sel2 : Selector  InputPortWidth=6  IndexOptions=Index vector (dialog)  Indices=[3 6]  OutputSizes=1
  ParasiticTo : Outport
  wires:
  Mux3/1 -> ParasiticTo/1
  Mux2/1 -> Sel/1, Sel2/1, Sel1/1
  MotTo/1 -> Mux2/1
  MotPos/1 -> Mux2/2
  Sel/1 -> Demux3/1
  Demux3/2 -> Parasitic AZ/2(MotPos)
  Parasitic AZ/1(To) -> Mux3/1
  Sel1/1 -> Demux1/1
  Demux1/2 -> Parasitic EL/2(MotPos)
  Parasitic EL/1(To) -> Mux3/2
  Demux2/1 -> Parasitic GIR/1(MotTo)
  Demux2/2 -> Parasitic GIR/2(MotPos)
  Sel2/1 -> Demux2/1
  Demux3/1 -> Parasitic AZ/1(MotTo)
  Demux1/1 -> Parasitic EL/1(MotTo)
  Parasitic GIR/1(To) -> Mux3/3

== system ims_Build5pt1g_tj/Mount_Drv_PDR2021/ODC CT LUGRE Fr model/Friction/Friction Alt/g(v) ==
  v : Inport
  Enable : EnablePort
  Constant : Constant  Value=0
  Sum : Sum  Inputs=|++
  gc : Constant  Value=Tc/sigma0
  gs : Subsystem
  g : Outport
  wires:
  Sum/1 -> g/1
  v/1 -> gs/1(v)
  gs/1(gs(v)) -> Sum/1
  gc/1 -> Sum/2
  Constant/1 -> gs/Enable

== system ims_Build5pt1g_tj/Mount_Drv_PDR2021/ODC CT LUGRE Fr model/Friction/Friction Alt/v2z ==
  v : Inport
  g(v) : Inport  Port=2
  z : Inport  Port=3
  Enable : EnablePort
  Abs : Abs
  Divide : Product  Inputs=*/*
  Sum : Sum  Inputs=|+-
  dz : Outport
  wires:
  Abs/1 -> Divide/1
  Divide/1 -> Sum/2
  v/1 -> Sum/1, Abs/1
  Sum/1 -> dz/1
  g(v)/1 -> Divide/2
  z/1 -> Divide/3

== system ims_Build5pt1g_tj/Mount_Drv_PDR2021/ODC CT LUGRE Fr model/Friction/Friction Az/g(v) ==
  v : Inport
  Enable : EnablePort
  Constant : Constant  Value=0
  Sum : Sum  Inputs=|++
  gc : Constant  Value=Tc/sigma0
  gs : Subsystem
  g : Outport
  wires:
  Sum/1 -> g/1
  v/1 -> gs/1(v)
  gs/1(gs(v)) -> Sum/1
  gc/1 -> Sum/2
  Constant/1 -> gs/Enable

== system ims_Build5pt1g_tj/Mount_Drv_PDR2021/ODC CT LUGRE Fr model/Friction/Friction Az/v2z ==
  v : Inport
  g(v) : Inport  Port=2
  z : Inport  Port=3
  Enable : EnablePort
  Abs : Abs
  Divide : Product  Inputs=*/*
  Sum : Sum  Inputs=|+-
  dz : Outport
  wires:
  Abs/1 -> Divide/1
  Divide/1 -> Sum/2
  v/1 -> Sum/1, Abs/1
  Sum/1 -> dz/1
  g(v)/1 -> Divide/2
  z/1 -> Divide/3

== system ims_Build5pt1g_tj/Mount_Drv_PDR2021/ODC CT LUGRE Fr model/Friction/Friction Gir/g(v) ==
  v : Inport
  Constant : Constant  Value=0
  Sum : Sum  Inputs=|++
  gc : Constant  Value=Tc/sigma0
  gs : Subsystem
  g : Outport
  wires:
  Sum/1 -> g/1
  v/1 -> gs/1(v)
  gs/1(gs(v)) -> Sum/1
  gc/1 -> Sum/2
  Constant/1 -> gs/Enable

== system ims_Build5pt1g_tj/Mount_Drv_PDR2021/ODC CT LUGRE Fr model/Friction/Friction Gir/v2z ==
  v : Inport
  g(v) : Inport  Port=2
  z : Inport  Port=3
  Abs : Abs
  Divide : Product  Inputs=*/*
  Sum : Sum  Inputs=|+-
  dz : Outport
  wires:
  Abs/1 -> Divide/1
  Divide/1 -> Sum/2
  v/1 -> Sum/1, Abs/1
  Sum/1 -> dz/1
  g(v)/1 -> Divide/2
  z/1 -> Divide/3

== system ims_Build5pt1g_tj/Mount_Drv_PDR2021/Parasitic torques model /Subsystem/Parasitic Torques/Parasitic AZ ==
  MotTo : Inport
  MotPos : Inport  Port=2
  Cogging : Lookup_n-D  NumberOfTableDimensions=1  LookupTableObject=F_ripple  BreakpointsForDimension1=Pos  Table=Amp_Cog  InternalRulePriority=Speed  RndMeth=Simplest  InputSameDT=on
  Constant : Constant  Value=0.1869
  Divide : Product  Inputs=**
  EMF Distortion : Lookup_n-D  NumberOfTableDimensions=1  LookupTableObject=F_ripple  BreakpointsForDimension1=Pos  Table=Amp_EMF  InternalRulePriority=Speed  RndMeth=Simplest  InputSameDT=on
  Gain : Gain  Gain=1/R
  Gain1 : Gain  Gain=1/250
  Gain2 : Gain  Gain=1/N_Segm
  Mod : Math  Operator=rem  SignedPower=on  SaturateOnIntegerOverflow=on
  Mod1 : Math  Operator=rem  SignedPower=on  SaturateOnIntegerOverflow=on
  Radius : Gain  Gain=R
  Sum : Sum  Inputs=|++
  Sum1 : Sum  Inputs=|++
  To : Outport
  wires:
  Radius/1 -> Mod/1  "driven  distance"
  Constant/1 -> Mod1/2, Sum1/2, Mod/2
  MotPos/1 -> Radius/1
  Sum/1 -> To/1
  Cogging/1 -> Sum/2
  MotTo/1 -> Gain/1
  Gain/1 -> Gain1/1  "Force"
  EMF Distortion/1 -> Divide/2
  Divide/1 -> Sum/1
  Gain2/1 -> Divide/1  "I_rms pro Segment"
  Gain1/1 -> Gain2/1  "I_rms"
  Mod/1 -> Sum1/1
  Sum1/1 -> Mod1/1
  Mod1/1 -> EMF Distortion/1, Cogging/1

== system ims_Build5pt1g_tj/Mount_Drv_PDR2021/Parasitic torques model /Subsystem/Parasitic Torques/Parasitic EL ==
  MotTo : Inport
  MotPos : Inport  Port=2
  Cogging : Lookup_n-D  NumberOfTableDimensions=1  LookupTableObject=F_ripple  BreakpointsForDimension1=Pos  Table=Amp_Cog  InternalRulePriority=Speed  RndMeth=Simplest  InputSameDT=on
  Constant : Constant  Value=0.1869
  Divide : Product  Inputs=**
  EMF Distortion : Lookup_n-D  NumberOfTableDimensions=1  LookupTableObject=F_ripple  BreakpointsForDimension1=Pos  Table=Amp_EMF  InternalRulePriority=Speed  RndMeth=Simplest  InputSameDT=on
  Gain : Gain  Gain=1/R
  Gain1 : Gain  Gain=1/250
  Gain2 : Gain  Gain=1/N_Segm
  Mod1 : Math  Operator=rem  SignedPower=on  SaturateOnIntegerOverflow=on
  Mod2 : Math  Operator=rem  SignedPower=on  SaturateOnIntegerOverflow=on
  Radius : Gain  Gain=R
  Scope : Scope  Commented=on  NumInputPorts=2
  Sum : Sum  Inputs=|++
  Sum1 : Sum  Inputs=|++
  To : Outport
  wires:
  MotPos/1 -> Radius/1
  Sum/1 -> To/1
  Cogging/1 -> Scope/2, Sum/2
  MotTo/1 -> Gain/1
  Gain/1 -> Gain1/1  "Force"
  EMF Distortion/1 -> Divide/2
  Divide/1 -> Scope/1, Sum/1
  Gain2/1 -> Divide/1  "I_rms pro Segment"
  Gain1/1 -> Gain2/1  "I_rms"
  Sum1/1 -> Mod2/1
  Mod1/1 -> Sum1/1
  Radius/1 -> Mod1/1  "driven distance"
  Constant/1 -> Mod2/2, Sum1/2, Mod1/2
  Mod2/1 -> Cogging/1, EMF Distortion/1

== system ims_Build5pt1g_tj/Mount_Drv_PDR2021/Parasitic torques model /Subsystem/Parasitic Torques/Parasitic GIR ==
  MotTo : Inport
  MotPos : Inport  Port=2
  Cogging : Subsystem
  Emf : Subsystem
  Pretention : Constant  Value=T_pretension
  Product2 : Product  RndMeth=Zero
  Scope : Scope  Commented=on  NumInputPorts=2
  Sign : Signum  ZeroCross=off
  Sum1 : Sum  Inputs=|++
  Sum2 : Sum  Inputs=++|
  To : Outport
  wires:
  Sum2/1 -> To/1
  MotPos/1 -> Cogging/1(Po), Emf/2(Po)
  Cogging/1(T_cog) -> Sum2/2
  Emf/1(T_emf) -> Sum2/1
  Sum1/1 -> Emf/1(To)
  Sign/1 -> Product2/1
  Pretention/1 -> Product2/2
  Product2/1 -> Sum1/2
  MotTo/1 -> Sign/1, Sum1/1

== system ims_Build5pt1g_tj/Mount_Drv_PDR2021/ODC CT LUGRE Fr model/Friction/Friction Alt/g(v)/gs ==
  v : Inport
  Enable : EnablePort
  Divide : Product  Inputs=**
  Gain : Gain  Gain=1/vs
  Math Function : Math  SignedPower=on  SaturateOnIntegerOverflow=on
  Math Function1 : Math  Operator=magnitude^2  SignedPower=on  SaturateOnIntegerOverflow=on
  Unary Minus : UnaryMinus
  gs : Constant  Value=(Ts-Tc)/sigma0
  gs(v) : Outport
  wires:
  Math Function/1 -> Divide/1
  gs/1 -> Divide/2
  Math Function1/1 -> Unary Minus/1
  Unary Minus/1 -> Math Function/1
  Gain/1 -> Math Function1/1
  v/1 -> Gain/1
  Divide/1 -> gs(v)/1

== system ims_Build5pt1g_tj/Mount_Drv_PDR2021/ODC CT LUGRE Fr model/Friction/Friction Az/g(v)/gs ==
  v : Inport
  Enable : EnablePort
  Divide : Product  Inputs=**
  Gain : Gain  Gain=1/vs
  Math Function : Math  SignedPower=on  SaturateOnIntegerOverflow=on
  Math Function1 : Math  Operator=magnitude^2  SignedPower=on  SaturateOnIntegerOverflow=on
  Unary Minus : UnaryMinus
  gs : Constant  Value=(Ts-Tc)/sigma0
  gs(v) : Outport
  wires:
  Math Function/1 -> Divide/1
  gs/1 -> Divide/2
  Math Function1/1 -> Unary Minus/1
  Unary Minus/1 -> Math Function/1
  Gain/1 -> Math Function1/1
  v/1 -> Gain/1
  Divide/1 -> gs(v)/1

== system ims_Build5pt1g_tj/Mount_Drv_PDR2021/ODC CT LUGRE Fr model/Friction/Friction Gir/g(v)/gs ==
  v : Inport
  Enable : EnablePort
  Divide : Product  Inputs=**
  Gain : Gain  Gain=1/vs
  Math Function : Math  SignedPower=on  SaturateOnIntegerOverflow=on
  Math Function1 : Math  Operator=magnitude^2  SignedPower=on  SaturateOnIntegerOverflow=on
  Unary Minus : UnaryMinus
  gs : Constant  Value=(Ts-Tc)/sigma0
  gs(v) : Outport
  wires:
  Math Function/1 -> Divide/1
  gs/1 -> Divide/2
  Math Function1/1 -> Unary Minus/1
  Unary Minus/1 -> Math Function/1
  Gain/1 -> Math Function1/1
  v/1 -> Gain/1
  Divide/1 -> gs(v)/1

== system ims_Build5pt1g_tj/Mount_Drv_PDR2021/Parasitic torques model /Subsystem/Parasitic Torques/Parasitic GIR/Cogging ==
  Po : Inport
  CogAmp : Constant  Value=cog_amp
  CogSpatFreq : Constant  Value=cog_sfr
  Product1 : Product  RndMeth=Zero
  Product2 : Product  RndMeth=Zero
  Trigonometric Function : Trigonometry
  T_cog : Outport
  wires:
  Product1/1 -> Trigonometric Function/1
  CogSpatFreq/1 -> Product1/2
  CogAmp/1 -> Product2/2
  Trigonometric Function/1 -> Product2/1
  Po/1 -> Product1/1
  Product2/1 -> T_cog/1

== system ims_Build5pt1g_tj/Mount_Drv_PDR2021/Parasitic torques model /Subsystem/Parasitic Torques/Parasitic GIR/Emf ==
  To : Inport
  Po : Inport  Port=2
  EmfAmpFactor : Constant  Value=emf_ampFact
  EmfSpatFreq : Constant  Value=emf_sfr
  Product1 : Product  RndMeth=Zero
  Product2 : Product  Inputs=3  RndMeth=Zero
  Trigonometric Function : Trigonometry
  T_emf : Outport
  wires:
  Product1/1 -> Trigonometric Function/1
  EmfSpatFreq/1 -> Product1/2
  EmfAmpFactor/1 -> Product2/2
  Trigonometric Function/1 -> Product2/1
  Po/1 -> Product1/1
  Product2/1 -> T_emf/1
  To/1 -> Product2/3
